simulink model "tp235580"  (Simulink 3.0)
settings: Solver=ode45  StartTime=0.0  StopTime=10.0  MaxStep=1e-3  RelTol=1e-6  AbsTol=1e-6
undefined symbols (not defined in the file): p0, v0, w0
libraries: simulink_extras x2
settings Model: LastModifiedBy=campa  SaveFormat=Matrix  BooleanDataType=on

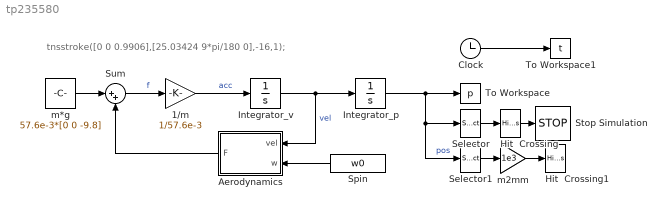
== system tp235580 ==
  note: tnsstroke([0 0 0.9906],[25.03424 9*pi/180 0],-16,1);
  1/m : Gain  Gain=1/57.6e-3  SaturateOnIntegerOverflow=on
  Aerodynamics : Subsystem  Orientation=left  mask(Ball Aerodynamics){R=32.5e-3, CD=0.48, CL=0.017, rho=1.229}
      mask prompts: R "Ball Radius (m)"; CD "Ball Drag Coefficient"; CL "Ball Lift Coefficient"; rho "Air Density (Kg/m^3)"
      mask help:
      | Computes aerodynamic forces on the tennis ball
      |    from linear and angular velocity. Ball characteristics
      |    and air density are taken as mask parameters.
      mask Help:
      | Computes aerodynamic forces on the tennis ball
      |    from linear and angular velocity. Ball characteristics
      |    and air density are taken as mask parameters.
  Clock : Clock
      settings: DisplayTime=off  Decimation=10
  Hit  Crossing : HitCross  HitCrossingOffset=0  HitCrossingDirection=either  ShowOutputPort=on
  Hit  Crossing1 : HitCross  HitCrossingOffset=23.7744/2  HitCrossingDirection=either  ShowOutputPort=off
  Integrator_p : Integrator  ExternalReset=none  InitialConditionSource=internal  InitialCondition=p0  LimitOutput=off  UpperSaturationLimit=inf  LowerSaturationLimit=-inf  ShowSaturationPort=off  ShowStatePort=off  AbsoluteTolerance=auto
  Integrator_v : Integrator  ExternalReset=none  InitialConditionSource=internal  InitialCondition=v0  LimitOutput=off  UpperSaturationLimit=inf  LowerSaturationLimit=-inf  ShowSaturationPort=off  ShowStatePort=off  AbsoluteTolerance=auto
  Selector : Selector  Elements=3  InputPortWidth=3
  Selector1 : Selector  Elements=1  InputPortWidth=3
  Spin : Constant  Orientation=left  Value=w0
  Stop Simulation : Stop
  Sum : Sum  Inputs=|++  SaturateOnIntegerOverflow=on
  To Workspace : ToWorkspace  VariableName=p  SampleTime=-1  SaveFormat=Matrix
  To Workspace1 : ToWorkspace  VariableName=t  SampleTime=-1  SaveFormat=Matrix
  m*g : Constant  Value=57.6e-3*[0 0 -9.8]
  m2mm : Gain  Gain=1e3  SaturateOnIntegerOverflow=on
  wires:
  Integrator_p/1 -> To Workspace/1, Selector/1, Selector1/1  "pos"
  Integrator_v/1 -> Integrator_p/1, Aerodynamics/1(vel)  "vel"
  Sum/1 -> 1/m/1  "f"
  Aerodynamics/1(F) -> Sum/2
  m*g/1 -> Sum/1
  Clock/1 -> To Workspace1/1
  Hit  Crossing/1 -> Stop Simulation/1
  Selector/1 -> Hit  Crossing/1
  1/m/1 -> Integrator_v/1  "acc"
  Spin/1 -> Aerodynamics/2(w)
  Selector1/1 -> m2mm/1
  m2mm/1 -> Hit  Crossing1/1

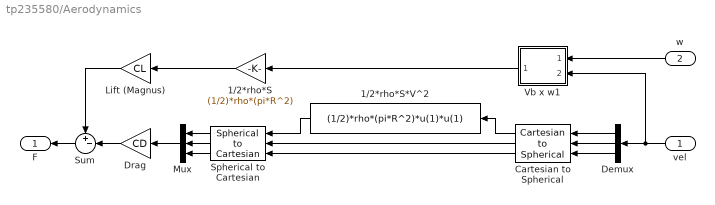
== system tp235580/Aerodynamics ==
  vel : Inport  Orientation=left  Port=1  PortWidth=-1  SampleTime=-1  DataType=auto
      settings: SignalType=auto
  w : Inport  Orientation=left  Port=2  PortWidth=-1  SampleTime=-1  DataType=auto
      settings: SignalType=auto
  1/2*rho*S : Gain  Orientation=left  Gain=(1/2)*rho*(pi*R^2)  SaturateOnIntegerOverflow=on
  1/2*rho*S*V^2 : Fcn  Orientation=left  Expr=(1/2)*rho*(pi*R^2)*u(1)*u(1)
  Cartesian to Spherical : simulink_extras/Transformations/Cartesian to Spherical  Orientation=left
  Demux : Demux  Orientation=left  Outputs=3
  Drag : Gain  Orientation=left  Gain=CD  SaturateOnIntegerOverflow=on
  Lift (Magnus) : Gain  Orientation=left  Gain=CL  SaturateOnIntegerOverflow=on
  Mux : Mux  Orientation=left  Inputs=3
  Spherical to Cartesian : simulink_extras/Transformations/Spherical to Cartesian  Orientation=left
  Sum : Sum  Orientation=left  Inputs=+-|  SaturateOnIntegerOverflow=on
  Vb x w1 : Subsystem  Orientation=left
      mask Type: Cross Product
      mask Description: Calculates the cross product of two 3x1 vectors.
      mask Help:
      | <p>This block calculates the cross product of two 3x1 vectors, ie.</p>
      | 
      | <ul>C(1) = A(2)*B(3) - A(3)*B(2)</ul>
      | <ul>C(2) = A(3)*B(1) - A(1)*B(3)</ul>
      | <ul>C(3) = A(1)*B(2) - A(2)*B(1)</ul>
      | 
      | <p>The block inputs and output contain more than one signal as described below.</p>
      | 
      | <p><H4>Block Vector Input 1 - A</H4>
      | <ul>
      | <li>A(1)</li>
      | <li>A(2)</li>
      | <li>A(3)</li>
      | </ul>
      | </p>
      | 
      | <p><H4>Block Vector Input 2 - B</H4>
      | <ul>
      | <li>B(1)</li>
      | <li>B(2)</li>
      | <li>B(3)</li>
      | </ul>
      | </p>
      | 
      | <p><H4>Block Vector Output - Cross Product (AxB)</H4>
      | <ul>
      | <li>C(1)</li>
      | <li>C(2)</li>
      | <li>C(3)</li>
      | </ul>
      | </p>
      mask Display: disp('Cross\nProduct')
  F : Outport  Orientation=left  Port=1
  wires:
  Demux/1 -> Cartesian to Spherical/1
  Demux/2 -> Cartesian to Spherical/2
  Demux/3 -> Cartesian to Spherical/3
  vel/1 -> Demux/1, Vb x w1/2(b(1) b(2) b(3))
  Cartesian to Spherical/1 -> 1/2*rho*S*V^2/1
  1/2*rho*S*V^2/1 -> Spherical to Cartesian/1
  Spherical to Cartesian/1 -> Mux/1
  Spherical to Cartesian/2 -> Mux/2
  Spherical to Cartesian/3 -> Mux/3
  Mux/1 -> Drag/1
  Cartesian to Spherical/2 -> Spherical to Cartesian/2
  Cartesian to Spherical/3 -> Spherical to Cartesian/3
  Vb x w1/1(c(1) c(2) c(3)) -> 1/2*rho*S/1
  Sum/1 -> F/1
  1/2*rho*S/1 -> Lift (Magnus)/1
  w/1 -> Vb x w1/1(a(1) a(2) a(3))
  Drag/1 -> Sum/2
  Lift (Magnus)/1 -> Sum/1

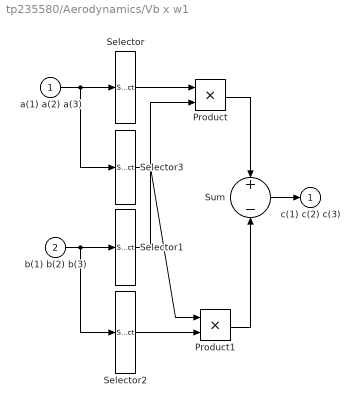
== system tp235580/Aerodynamics/Vb x w1 ==
  a(1) a(2) a(3) : Inport  Port=1  PortWidth=-1  SampleTime=-1  DataType=auto
      settings: SignalType=auto
  b(1) b(2) b(3) : Inport  Port=2  PortWidth=-1  SampleTime=-1  DataType=auto
      settings: SignalType=auto
  Product : Product  Inputs=2  SaturateOnIntegerOverflow=on
  Product1 : Product  Inputs=2  SaturateOnIntegerOverflow=on
  Selector : Selector  Elements=[2 3 1]  InputPortWidth=3
  Selector1 : Selector  Elements=[3 1 2]  InputPortWidth=3
  Selector2 : Selector  Elements=[2 3 1]  InputPortWidth=3
  Selector3 : Selector  Elements=[3 1 2]  InputPortWidth=3
  Sum : Sum  Inputs=+|-  SaturateOnIntegerOverflow=on
  c(1) c(2) c(3) : Outport  Port=1  InitialOutput=0
  wires:
  Sum/1 -> c(1) c(2) c(3)/1
  b(1) b(2) b(3)/1 -> Selector1/1, Selector2/1
  Selector/1 -> Product/1
  a(1) a(2) a(3)/1 -> Selector/1, Selector3/1
  Product/1 -> Sum/1
  Selector1/1 -> Product/2
  Product1/1 -> Sum/2
  Selector2/1 -> Product1/2
  Selector3/1 -> Product1/1
